simulink model "zero_relative_v_high_gap"  (R2025a)
settings: Solver=VariableStepAuto  StartTime=0.0  StopTime=10.0  RelTol=1e-3
settings Model: Creator=sanborkl  LastModifiedBy=sanborkl

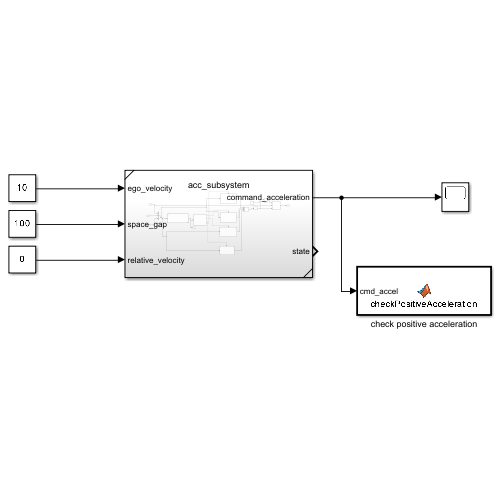
[thumbnail: Simulink's stored preview of the top-level diagram]
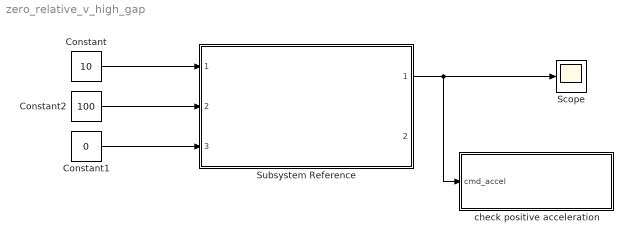
== system zero_relative_v_high_gap ==
  Constant : Constant  Value=10
  Constant1 : Constant  Value=0
  Constant2 : Constant  Value=100
  Scope : Scope
      settings: ActiveDisplayYMinimum=0.5  ActiveDisplayYMaximum=2.5
  Subsystem Reference : Subsystem  ReferencedSubsystem=acc_subsystem
  check positive acceleration : MATLAB Function  TreatAsAtomicUnit=on
  wires:
  Subsystem Reference/1 -> check positive acceleration/1(cmd_accel), Scope/1
  Constant/1 -> Subsystem Reference/1
  Constant1/1 -> Subsystem Reference/3
  Constant2/1 -> Subsystem Reference/2

== matlab function zero_relative_v_high_gap/check positive acceleration ==
  data: cmd_accel input
function checkPositiveAcceleration(cmd_accel)
%#codegen
coder.extrinsic('disp', 'sprintf');

if cmd_accel < 0
    msg = sprintf('Error: Negative command acceleration: %.3f, should be positive', ...
                  cmd_accel);
    disp(msg);
end
end
